simulink model "pci1756a"  (R2016b)
settings: Solver=ode4  StartTime=0.0  StopTime=inf  FixedStep=0.002  RelTol=1e-3  EnableMultiTasking=on
settings Model: SimulationMode=external  Creator=Administrator  LastModifiedBy=Administrator
settings SolverCC: EnableConcurrentExecution=on
settings DataIOCC: SaveFormat=StructureWithTime
settings OptimizationCC: BlockReduction=off  OptimizeBlockIOStorage=off  BufferReuse=off  GlobalBufferReuse=off  ExpressionFolding=off  LocalBlockOutputs=off
settings HardwareCC: ProdBitPerPointer=32  ProdBitPerSizeT=32  ProdBitPerPtrDiffT=32  ProdLargestAtomicFloat=None  ProdWordSize=32  ProdLongLongMode=on  ProdHWDeviceType=Generic->32-bit x86 compatible
settings RTWCC: SystemTargetFile=slrt.tlc  TemplateMakefile=slrt_default_tmf  Description=Simulink Real-Time  RTWCompilerOptimization=on

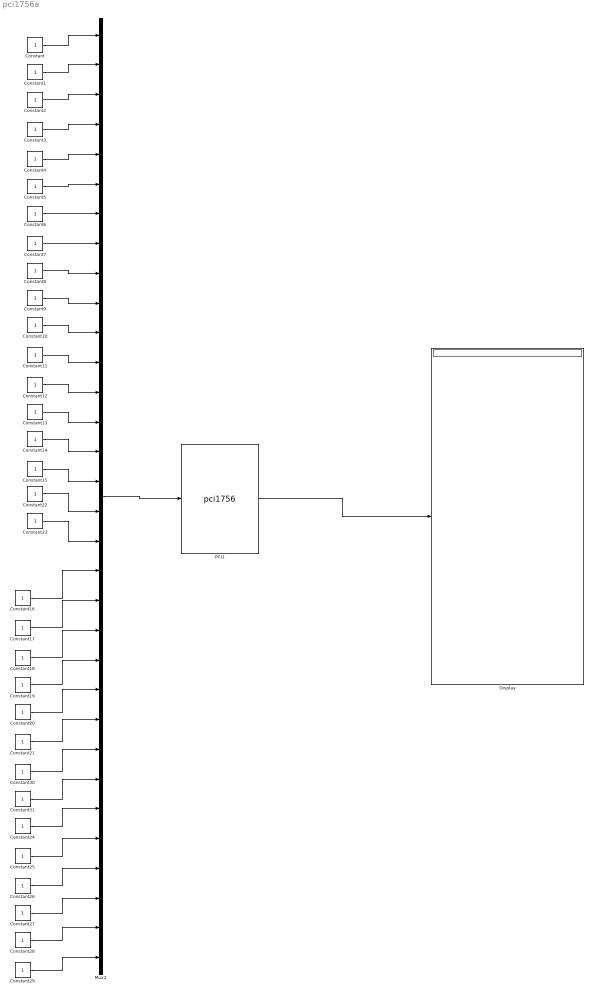
== system pci1756a ==
  Constant{,1..31} (32 alike) : Constant
  Display : Display
  Mux2 : Mux  Inputs=32
  PCI1 : S-Function  FunctionName=pci1756  Parameters=BaseAddress, [SampleTime SampleOffset]  SFunctionDeploymentMode=off  EnableBusSupport=off  mask(PCI1756){sBaseAddr=0xe, Sample=0.002}
      mask prompts: sBaseAddr "PCI_1756 ADRESS :"; Sample "Sample Time:"
      mask help:
      | PCI-1756
      | Advantech
      | Digital Input&Output
      mask init:
      | BaseAddress = 0;SampleTime = 0.002; SampleOffset = 0;
      | sampleLength = length (Sample);
      | %if (sampleLength > 2)
      | %  error ('Sample length vector cannot exceed two elements');
      | %end
      | if (sampleLength == 2)
      |   SampleTime = Sample(1);
      |   SampleOffset = Sample(2);
      | else
      |   SampleTime = Sample(1);
      |   SampleOffset = 0;
      | end
      | 
      | sBaseAddr(find(sBaseAddr=='''')) = [];
      | index = findstr(lower(sBaseAddr),'0x');
      | if ~isempty(index) & index==1
      |   BaseAddr = sBaseAddr(3:end);
      |   baLength = length (BaseAddr);
      |   baseStringMember = [abs('0'):abs('9'),abs('a'):abs('f'),abs('A'):abs('F')];
      |   for i = 1:baLength
      |  %   if ~ismember(BaseAddr(i),baseStringMember)
      |  %     error ('Invalid character in hexadecimal string');
      |  %   end
      |   end
      |   BaseAddress = hex2dec(BaseAddr);
      | else
      |   BaseAddrress = str2num(BaseAddr);
      | end
      mask Display:
      | fprintf('PCI1756\n\nSample time:\n%g\nBaseAdress:\n%s', Sample,sBaseAddr)
      | port_label('input',1,'32');
      | port_label('output',1,'32');
  wires:
  Constant/1 -> Mux2/1
  Constant1/1 -> Mux2/2
  Constant2/1 -> Mux2/3
  Constant3/1 -> Mux2/4
  Constant4/1 -> Mux2/5
  Constant5/1 -> Mux2/6
  Constant6/1 -> Mux2/7
  Constant7/1 -> Mux2/8
  Constant8/1 -> Mux2/9
  Constant9/1 -> Mux2/10
  Constant10/1 -> Mux2/11
  Constant11/1 -> Mux2/12
  Constant12/1 -> Mux2/13
  Constant13/1 -> Mux2/14
  Constant14/1 -> Mux2/15
  Constant15/1 -> Mux2/16
  Constant22/1 -> Mux2/17
  Constant23/1 -> Mux2/18
  Constant16/1 -> Mux2/19
  Constant17/1 -> Mux2/20
  Constant18/1 -> Mux2/21
  Constant19/1 -> Mux2/22
  Constant20/1 -> Mux2/23
  Constant21/1 -> Mux2/24
  Constant30/1 -> Mux2/25
  Constant31/1 -> Mux2/26
  Constant24/1 -> Mux2/27
  Constant25/1 -> Mux2/28
  Constant26/1 -> Mux2/29
  Constant27/1 -> Mux2/30
  Constant28/1 -> Mux2/31
  Constant29/1 -> Mux2/32
  Mux2/1 -> PCI1/1
  PCI1/1 -> Display/1
